simulink model "controller_dev_sg_HIL_noTP"  (R2018b)
settings: configuration reference "Physics" (kept outside this file)
model workspace (MAT data in the model file):
  m = 1000
values from neighbouring files (symbols this model uses):
  bool_activate_Vehicles : value not decoded    [controller_dev_sg.sldd]
  ModObj_ObjList_SendPort = 11004.0    [UDPPortConfig.sldd]
  ModSens_GpsSenDat_SendPort = 3002.0    [UDPPortConfig.sldd]
  sensors_freq_camera = 37.0    [controller_dev_sg.sldd]
  sensors_freq_gps = 20.0    [controller_dev_sg.sldd]
  sensors_freq_imu = 100.0    [controller_dev_sg.sldd]
  sensors_freq_lidar = 12.0    [controller_dev_sg.sldd]
  sensors_freq_radar = 20.0    [controller_dev_sg.sldd]
undefined symbols (not defined in the file or in its folder): activate_VariableFriction, C, tpa_map_Reference, tSPhysics, x0_vehiclepos_start_veh1, x0_vehiclepos_start_veh10, x0_vehiclepos_start_veh2, x0_vehiclepos_start_veh3, x0_vehiclepos_start_veh4, x0_vehiclepos_start_veh5, x0_vehiclepos_start_veh6, x0_vehiclepos_start_veh7, x0_vehiclepos_start_veh8, x0_vehiclepos_start_veh9
libraries: xpcutilitieslib x273, xpcrtudplib x215, aerolibconvert2 x48, simulink x30, etargetslib x26, speedgoatlib_IO612 x7, canmsglib x6, slrtlib x4
(part 16 of 16)

== matlab function controller_dev_sg_HIL_noTP/UDP to Sensors (GNSS, IMU)7/DUALANTENNAHEADING/CRC1 ==
  data: data input; crc output
function crc = fcn(data)

crc = crc32(data);

== matlab function controller_dev_sg_HIL_noTP/UDP to Sensors (GNSS, IMU)7/DUALANTENNAHEADING/Header1 ==
  data: id input; first output; length input; time input; leapseconds input; second output; third output; hlength output; id output; type output; port output; mlength output; seq output; idletime output; timestatus output; week output; ms output; recstatus output; reserved output; version output
function [first, second, third, hlength, id, type, port, mlength, seq, idletime, timestatus, week, ms, recstatus, reserved, version] = fcn(id, length, time, leapseconds)

[first, second, third, hlength, id, type, port, mlength, seq, idletime, timestatus, week, ms, recstatus, reserved, version] = novatel_header(id, length, time, leapseconds);

== matlab function controller_dev_sg_HIL_noTP/UDP to Sensors (GNSS, IMU)7/DUALANTENNAHEADING/grid conv angle1 ==
  data: lat input; gamma output; lon input
function gamma = fcn(lat, lon)

gamma = grid_conv_angle(lat, lon);

== matlab function controller_dev_sg_HIL_noTP/UDP to Sensors (GNSS, IMU)7/DUALANTENNAHEADING/normalizeAngle1 ==
  data: u input; y output
function y = fcn(u)

y = normalizeAngle360(u);

== matlab function controller_dev_sg_HIL_noTP/UDP to Sensors (GNSS, IMU)7/DUALANTENNAHEADING/tcs2llhT1 ==
  data: x input; lat output; y input; z input; origin input; lon output; hgt output
function [lat, lon, hgt]= fcn(x, y, z, origin)

llh =tcs2llhT([x; y; z], origin);
lat = llh(1,:);
lon = llh(2,:);
hgt = llh(3,:);
end
